simulink model "robot_arm_1_dof"  (R2023a)
settings: Solver=ode14x  StartTime=0.0  StopTime=10  FixedStep=0.1  RelTol=1e-3  EnableMultiTasking=on
libraries: simulink_extras x1
settings Model: Creator=suteo  LastModifiedBy=ninju
settings SolverCC: AlgebraicLoopSolver=TrustRegion
settings DataIOCC: LimitDataPoints=on  SaveFormat=Array  ReturnWorkspaceOutputs=off
settings OptimizationCC: LifeSpan=inf
settings DebuggingCC: UnconnectedInputMsg=warning  UnconnectedOutputMsg=warning  UnconnectedLineMsg=warning  SFUnexpectedBacktrackingDiag=warning  SFNoUnconditionalDefaultTransitionDiag=warning  SFExecutionAtInitializationDiag=none  ArithmeticOperatorsInVariantConditions=warning
settings HardwareCC: ProdBitPerPointer=32  ProdBitPerSizeT=32  ProdBitPerPtrDiffT=32  ProdLargestAtomicFloat=None  ProdIntDivRoundTo=Undefined  ProdEndianess=Unspecified  ProdWordSize=32  ProdHWDeviceType=32-bit Generic
settings ModelReferenceCC: EnableRefExpFcnMdlSchedulingChecks=on  PropagateSignalLabelsOutOfModel=off
settings SFSimCC: SimUseLocalCustomCode=off  CustomCodeUndefinedFunction=UseInterfaceOnly
settings RTWCC: RTWUseLocalCustomCode=off
settings CodeAppCC: StateflowObjectComments=on
settings GRTTargetCC: TargetLangStandard=C89/C90 (ANSI)
settings ConfigComp: CovMetricSettings=dw  CovSaveCumulativeToWorkspaceVar=on  CovSaveSingleToWorkspaceVar=on  CovExternalEMLEnable=off  CovSFcnEnable=off

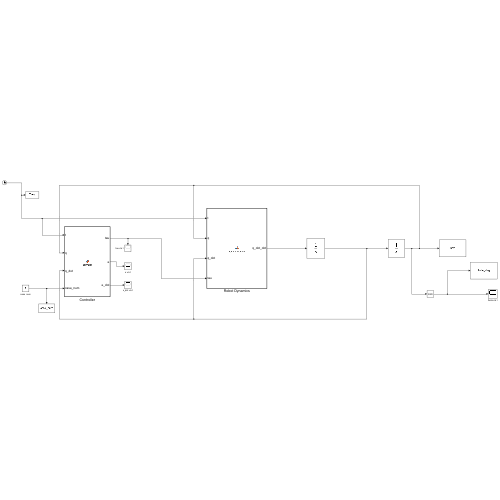
[thumbnail: Simulink's stored preview of the top-level diagram]
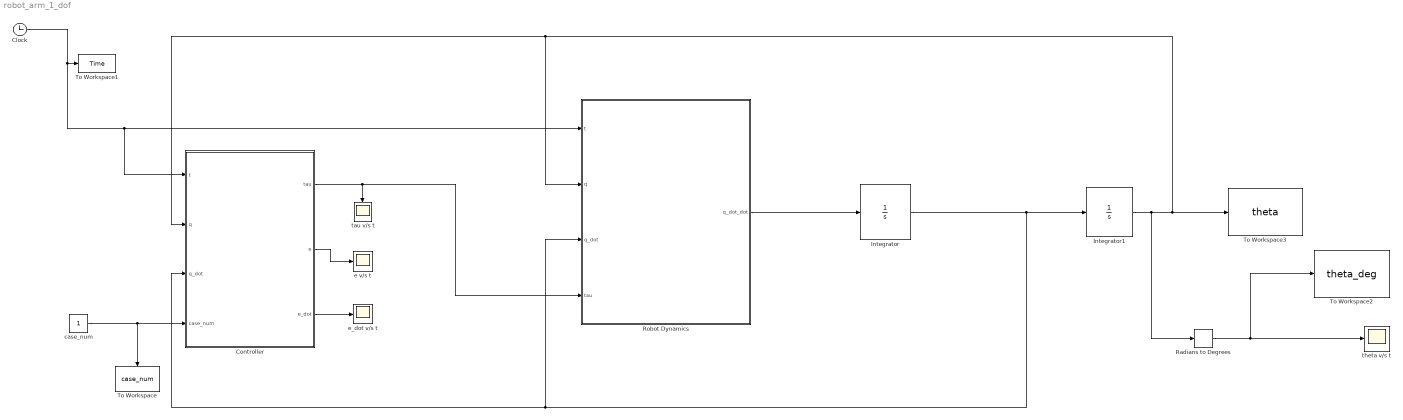
== system robot_arm_1_dof ==
  Clock : Clock
  Controller : MATLAB Function  TreatAsAtomicUnit=on
  Integrator : Integrator  InitialCondition=[0; 0]
  Integrator1 : Integrator  InitialCondition=[0; 0]
  Radians to Degrees : simulink_extras/Transformations/Radians to Degrees
  Robot Dynamics : MATLAB Function  TreatAsAtomicUnit=on
  To Workspace : ToWorkspace  VariableName=case_num  SampleTime=-1
      settings: Save2DSignal=2-D array (concatenate along first dimension)
  To Workspace1 : ToWorkspace  VariableName=Time  SampleTime=-1
  To Workspace2 : ToWorkspace  VariableName=theta_deg  SampleTime=-1
  To Workspace3 : ToWorkspace  VariableName=theta  SampleTime=-1
  case_num : Constant
  e v/s t : Scope
  e_dot v/s t : Scope
  tau v/s t : Scope
  theta v/s t : Scope
  wires:
  Clock/1 -> Controller/1(t), Robot Dynamics/1(t), To Workspace1/1
  Robot Dynamics/1(q_dot_dot) -> Integrator/1
  Integrator/1 -> Controller/3(q_dot), Robot Dynamics/3(q_dot), Integrator1/1
  Integrator1/1 -> Radians to Degrees/1, To Workspace3/1, Robot Dynamics/2(q), Controller/2(q)
  Controller/1(tau) -> Robot Dynamics/4(tau), tau v/s t/1
  Radians to Degrees/1 -> theta v/s t/1, To Workspace2/1
  case_num/1 -> Controller/4(case_num), To Workspace/1
  Controller/2(e) -> e v/s t/1
  Controller/3(e_dot) -> e_dot v/s t/1

== matlab function robot_arm_1_dof/Controller ==
  data: t input; tau output; q input; q_dot input; case_num input; e output; e_dot output
function [tau, e, e_dot] = controller(t, q, q_dot, case_num)

k= [1000;1000];

q_d=[pi/3; pi/4];
e = q - q_d; 
e_dot = q_dot;

if case_num == 1
    q_d=[(pi/4)*(sin(t)); (pi/5)*(cos(t))];
    q_d_dot = [(pi/4)*(cos(t)); -(pi/5)*(sin(t))];
    e = q - q_d;
    e_dot = q_dot - q_d_dot;
end

tau = -k(1)*e - k(2)*e_dot;

== matlab function robot_arm_1_dof/Robot Dynamics ==
  data: t input; q_dot_dot output size=2; q input; q_dot input; tau input
function q_dot_dot = robo_dynamics(t, q, q_dot, tau)

m1 = 1;
m2 = 1;
a1 = 1;
a2 = 1;
g = 10;

M = [[(m1 + m2)*a1^(2) + m2*a2^(2) + 2*m2*a1*a2*cos(q(2)), m2*a2^(2) + m2*a1*a2*cos(q(2))]; [m2*a2^(2) + m2*a1*a2*cos(q(2)), m2*a2^(2)]];

V = [-m2*a1*a2*(2*q_dot(1)*q_dot(2) + q_dot(2)^(2))*sin(q(2)); m2*a1*a2*q(1)^(2)*sin(q(2))];

G = [(m1+m2)*g*a1*cos(q(1)) + m2*g*a2*cos(q(1) + q(2)); m2*g*a2*cos(q(1) + q(2))];

q_dot_dot = inv(M) * (tau - G - V);
